simulink model "tstconvcod"  (Simulink 6.0)
settings: Solver=ode45  SolverMode=SingleTasking  StartTime=0.0  StopTime=Inf  RelTol=1e-3
undefined symbols (not defined in the file or in its folder): slcm
libraries: commcnvcod2 x2, commsequence2 x2, commchan2 x1, commdigbbndpm2 x1, commrandsrc2 x1, commsink2 x1
CloseFcn:
  | clear convSigsOut
settings Model: RequirementInfo=9  CovMetricSettings=d  Creator=mikem  LastModifiedBy=mmclerno  ExtModeTrigMode=oneshot  ExtModeArmWhenConnect=off
settings DataIOCC: LimitDataPoints=off  SaveOutput=off  SaveTime=off  SignalLoggingName=convSigsOut
settings OptimizationCC: BlockReduction=off  BooleanDataType=off  InlineInvariantSignals=off  MultiInstanced=off
settings FormatCC: IgnoreBidirectionalLines=off
settings DebuggingCC: IntegerOverflowMsg=none
settings HardwareCC: TargetUnknown=on
settings CodeAppCC: SimulinkBlockComments=off
settings GRTTargetCC: TargetFcnLib=iso_c_tmw.mat

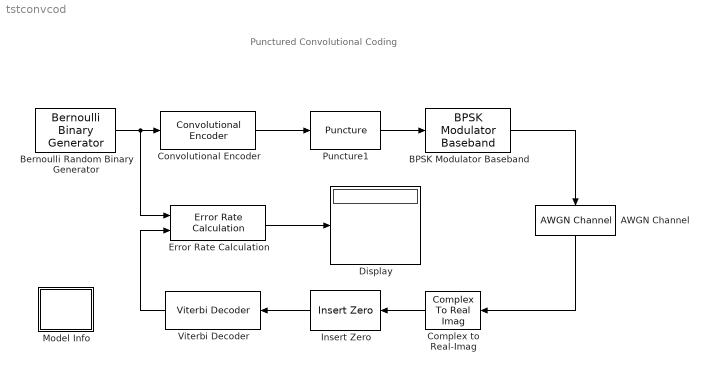
== system tstconvcod ==
  note: Punctured Convolutional Coding
  AWGN Channel : commchan2/AWGN Channel  Orientation=down  seed=123456  noiseMode="Signal to noise ratio  (Es/No)"  EbNodB=10  EsNodB=2  SNRdB=10  bitsPerSym=1  Ps=1  Tsym=0.75  variance=1
  BPSK Modulator Baseband : commdigbbndpm2/BPSK Modulator Baseband  Ph=0  numSamp=1
  Bernoulli Random Binary Generator : commrandsrc2/Bernoulli Binary Generator  P=0.5  seed=435345  Ts=1  frameBased=on  sampPerFrame=3  orient=off
  Complex to Real-Imag : ComplexToRealImag  Orientation=left  Output=Real
  Convolutional Encoder : commcnvcod2/Convolutional Encoder  trellis=poly2trellis(7, [171 133])  reset=None
  Display : Display
  Error Rate Calculation : commsink2/Error Rate Calculation  N=96  st_delay=0  cp_mode=Entire frame  subframe=[]  PMode=Port  WsName=BER_Data  RsMode2=off  stop=on  numErr=100  maxBits=1e6
  Insert Zero : commsequence2/Insert Zero  Orientation=left  insertZeroVector=[1 1 0 1 1 0].'
  Model Info : Subsystem  LoadFcn=slcm LoadBlock;  InitFcn=slcm('UpdateAllCMBlocksInThisModelInit')  mask(CMBlock){InitialSaveTempField=, InitialBlockCM=none, BlockCM=none, Frame=on, SaveTempField=, DisplayStringWithTags=Info, MaskDisplayString=Info, HorizontalTextAlignment=Center, LeftAlignmentValue=0.5, SourceBlockDiagram=tstconvcod, TagMaxNumber=20, CMTag1=, CMTag2=, CMTag3=, CMTag4=, CMTag5=, CMTag6=, CMTag7=, CMTag8=, CMTag9=, CMTag10=, CMTag11=, CMTag12=, CMTag13=, CMTag14=, CMTag15=, CMTag16=, CMTag17=, CMTag18=, CMTag19=, CMTag20=}
      mask help: This block allows revision control information to be displayed within the model.
      settings: CopyFcn=slcm CopyBlock;  DeleteFcn=slcm Cancel;  PostSaveFcn=slcm('UpdateAllCMBlocksInThisModel')  NameChangeFcn=slcm Rename;  OpenFcn=commdemohelp;
      mask Display: text(str2num(LeftAlignmentValue), 0.5, MaskDisplayString, 'HorizontalAlignment', HorizontalTextAlignment)
  Puncture1 : commsequence2/Puncture  punctureVector=[1 1 0 1 1 0].'
  Viterbi Decoder : commcnvcod2/Viterbi Decoder  Orientation=left  trellis=poly2trellis(7, [171 133])  dectype=Unquantized  nsdecb=4  tbdepth=96  opmode=Continuous  reset=off
  wires:
  Bernoulli Random Binary Generator/1 -> Convolutional Encoder/1, Error Rate Calculation/1
  Convolutional Encoder/1 -> Puncture1/1
  Puncture1/1 -> BPSK Modulator Baseband/1
  Insert Zero/1 -> Viterbi Decoder/1
  AWGN Channel/1 -> Complex to Real-Imag/1
  BPSK Modulator Baseband/1 -> AWGN Channel/1
  Complex to Real-Imag/1 -> Insert Zero/1
  Viterbi Decoder/1 -> Error Rate Calculation/2
  Error Rate Calculation/1 -> Display/1

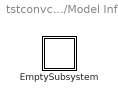
== system tstconvcod/Model Info ==
  EmptySubsystem : Subsystem

== system tstconvcod/Model Info/EmptySubsystem ==
